simulink model "Ex2"  (R2020a)
settings: Solver=VariableStepAuto  StartTime=0.0  StopTime=10.0  RelTol=1e-3

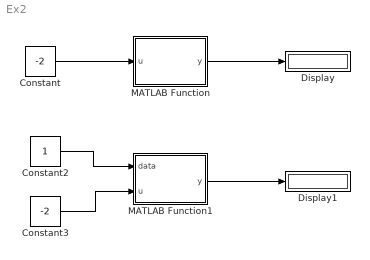
== system Ex2 ==
  Constant : Constant  Value=-2
  Constant2 : Constant
  Constant3 : Constant  Value=-2
  Display : Display
  Display1 : Display
  MATLAB Function : MATLAB Function  TreatAsAtomicUnit=on
  MATLAB Function1 : MATLAB Function  TreatAsAtomicUnit=on
  wires:
  Constant/1 -> MATLAB Function/1(u)
  MATLAB Function/1(y) -> Display/1
  Constant3/1 -> MATLAB Function1/2(u)
  Constant2/1 -> MATLAB Function1/1(data)
  MATLAB Function1/1(y) -> Display1/1

== matlab function Ex2/MATLAB Function ==
  data: u input; y output
function y = fcn(u)

  if u>=1 u=u*u;
      else  u=u*u*u;
  end

y = u;

== matlab function Ex2/MATLAB Function1 ==
  data: data input; u input; y output
function y  = fcn(data, u)

z=data+u;

if z<=2 && z>=0
    y=z*z;
    else y=data*data+u*u;
end

end
